simulink model "Receiver"  (R2021b)
settings: Solver=ode1  StartTime=0.0  StopTime=inf  FixedStep=0.001  RelTol=1e-3
settings Model: Creator=jalfonso  LastModifiedBy=au602135
settings SolverCC: AlgebraicLoopSolver=TrustRegion
settings DataIOCC: ReturnWorkspaceOutputs=off
settings DebuggingCC: SFMachineParentedDataDiag=warning  ArithmeticOperatorsInVariantConditions=warning
settings SFSimCC: SimUseLocalCustomCode=off  CustomCodeUndefinedFunction=UseInterfaceOnly
settings RTWCC: RTWUseLocalCustomCode=off
settings CodeAppCC: StateflowObjectComments=on

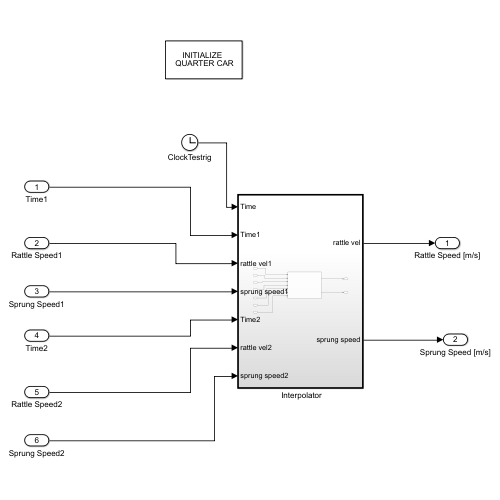
[thumbnail: Simulink's stored preview of the top-level diagram]
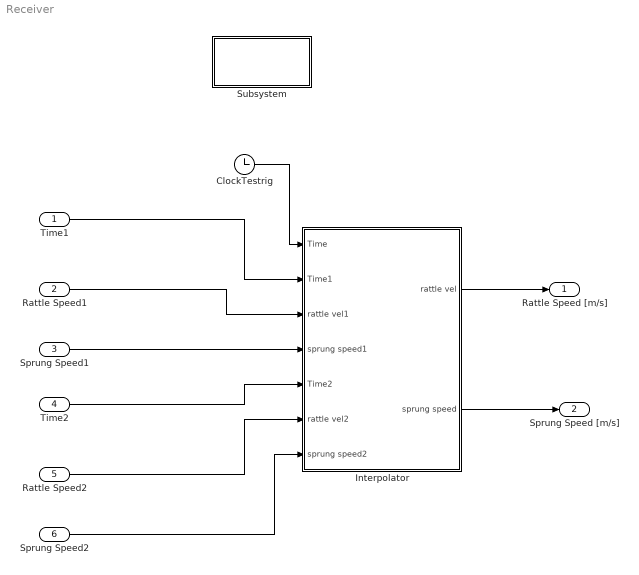
== system Receiver ==
  Time1 : Inport
  Rattle Speed1 : Inport  Port=2
  Sprung Speed1 : Inport  Port=3
  Time2 : Inport  Port=4
  Rattle Speed2 : Inport  Port=5
  Sprung Speed2 : Inport  Port=6
  " Interpolator" : Subsystem  TreatAsAtomicUnit=on
  ClockTestrig : Clock
  Subsystem : Subsystem
      settings: OpenFcn=|
      | k_tire = 225400;  %200000 in literature
      | c_tire = 100;        % Estimated. In literatures 6N
      | k_susp =  25000;  % 15000 in literature
      | c_susp = 400;       %1429 Ns/m in literature
      | g = 0 % 9.8; Removed to avoid initialization problems
      | m_unsprung = 66;
      | m_sprung = 449.25;
      | X_sprung0  = .5;
      | X_unsprung0  = .1;
      | delayTimeCarToDamper =  0.002;
      | %InitQuarterCarCompensatorScript;
      | %Amplitude =.01;
      mask Display: disp('INITIALIZE \n QUARTER CAR')
  Rattle Speed [m/s] : Outport
  Sprung Speed [m/s] : Outport  Port=2
  wires:
  Rattle Speed1/1 -> " Interpolator"/3(rattle vel1)
  Rattle Speed2/1 -> " Interpolator"/6(rattle vel2)
  Sprung Speed2/1 -> " Interpolator"/7(sprung speed2)
  Time2/1 -> " Interpolator"/5(Time2)
  Time1/1 -> " Interpolator"/2(Time1)
  " Interpolator"/1(rattle vel) -> Rattle Speed [m/s]/1
  ClockTestrig/1 -> " Interpolator"/1(Time)
  " Interpolator"/2(sprung speed) -> Sprung Speed [m/s]/1
  Sprung Speed1/1 -> " Interpolator"/4(sprung speed1)

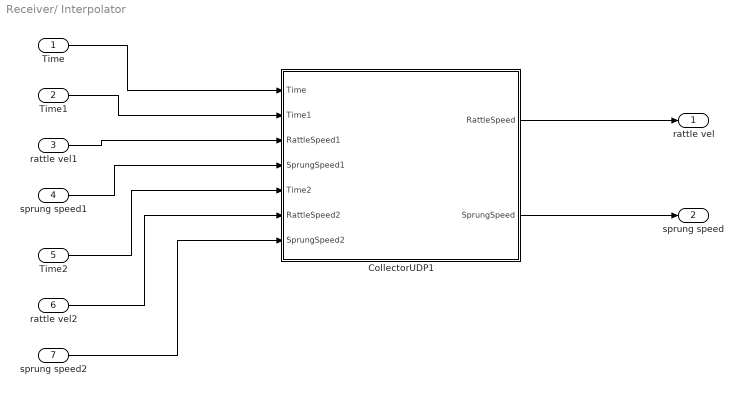
== system Receiver/ Interpolator ==
  Time : Inport
  Time1 : Inport  Port=2
  rattle vel1 : Inport  Port=3
  sprung speed1 : Inport  Port=4
  Time2 : Inport  Port=5
  rattle vel2 : Inport  Port=6
  sprung speed2 : Inport  Port=7
  CollectorUDP1 : MATLAB Function  TreatAsAtomicUnit=on
  rattle vel : Outport
  sprung speed : Outport  Port=2
  wires:
  sprung speed2/1 -> CollectorUDP1/7(SprungSpeed2)
  rattle vel1/1 -> CollectorUDP1/3(RattleSpeed1)
  Time1/1 -> CollectorUDP1/2(Time1)
  sprung speed1/1 -> CollectorUDP1/4(SprungSpeed1)
  Time/1 -> CollectorUDP1/1(Time)
  Time2/1 -> CollectorUDP1/5(Time2)
  rattle vel2/1 -> CollectorUDP1/6(RattleSpeed2)
  CollectorUDP1/2(SprungSpeed) -> sprung speed/1
  CollectorUDP1/1(RattleSpeed) -> rattle vel/1

== system Receiver/Subsystem ==

== matlab function Receiver/ Interpolator/CollectorUDP1 ==
  settings: updateMethod=DISCRETE
  data: Time input double; Time1 input double; RattleSpeed1 input double; RattleSpeed output double; SprungSpeed output double; SprungSpeed1 input double; Time2 input double; RattleSpeed2 input double; SprungSpeed2 input
function [RattleSpeed, SprungSpeed] = collectorInterpolator(Time, Time1, RattleSpeed1,SprungSpeed1,Time2, RattleSpeed2,SprungSpeed2)  

%initialization of buffer
persistent Buffer_Time1,persistent Buffer_RattleSpeed1,persistent Buffer_SprungSpeed1;
persistent Buffer_Time2,persistent Buffer_RattleSpeed2,persistent Buffer_SprungSpeed2;
if isempty(Buffer_Time1)  
   Buffer_Time1 = Time1;
   Buffer_RattleSpeed1 = RattleSpeed1;
   Buffer_SprungSpeed1 = SprungSpeed1;
   Buffer_Time2 = Time2;
   Buffer_RattleSpeed2 = RattleSpeed2;
   Buffer_SprungSpeed2 = SprungSpeed2;
end
%Buffer and message order check
if Time1 > Buffer_Time1
   Buffer_Time1 = Time1;
   Buffer_RattleSpeed1 = RattleSpeed1;
   Buffer_SprungSpeed1 = SprungSpeed1;
   Buffer_Time2 = Time2;
   Buffer_RattleSpeed2 = RattleSpeed2;
   Buffer_SprungSpeed2 = SprungSpeed2;
end

   
%Calculus of the current values based in linear interpolation
if (Buffer_Time2-Buffer_Time1)>0 
    RattleSpeed =  (Buffer_RattleSpeed2-Buffer_RattleSpeed1)/(Buffer_Time2-Buffer_Time1)*(Time-Buffer_Time1)+Buffer_RattleSpeed1;
    SprungSpeed =  (Buffer_SprungSpeed2-Buffer_SprungSpeed1)/(Buffer_Time2-Buffer_Time1)*(Time-Buffer_Time1)+Buffer_SprungSpeed1;
else
    RattleSpeed = 0;
    SprungSpeed = 0;
end
